simulink model "rigidBody2d"  (Simulink 7.5)
settings: Solver=ode45  StartTime=0.0  StopTime=40  RelTol=1e-3
undefined symbols (not defined in the file or in its folder): sigbuilder_block
settings Model: Creator=aaron  LastModifiedBy=aaron
settings DebuggingCC: SolverPrmCheckMsg=none

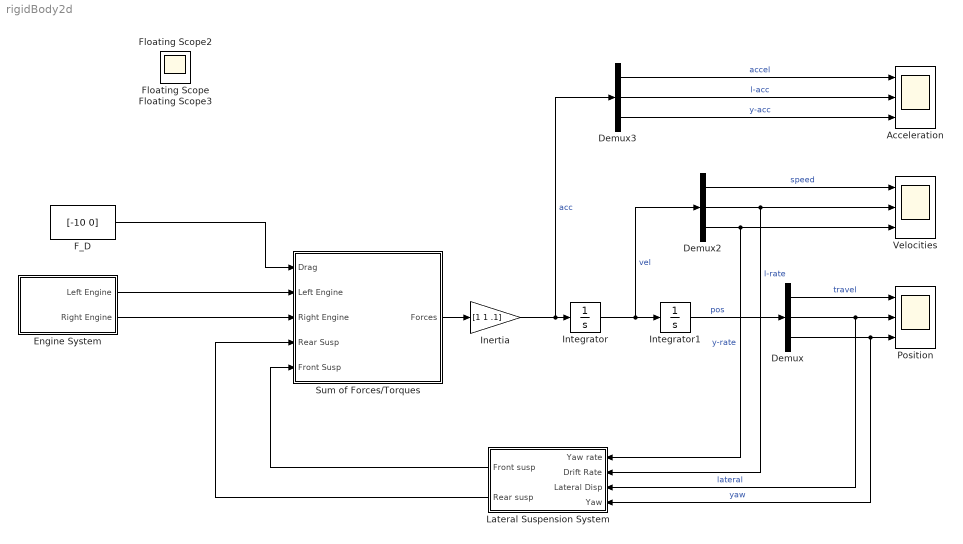
== system rigidBody2d ==
  Acceleration : Scope  NumInputPorts=3
      settings: YMin=-5~-5~-5  YMax=5~5~5  SaveName=position3
  Demux : Demux  Outputs=3
  Demux2 : Demux  Outputs=3
  Demux3 : Demux  Outputs=3
  Engine System : Subsystem
  F_D : Constant  Value=[-10 0]  OutDataType=fixdt(1, 16)  OutScaling=2^0
  Inertia : Gain  Gain=[1 1 .1]  ParameterDataType=fixdt(1, 16)  ParameterScaling=2^0  OutDataType=fixdt(1, 16)  OutScaling=2^0
  Integrator : Integrator  InitialCondition=[100 0 0]
  Integrator1 : Integrator  InitialCondition=[0 0 0]
  Lateral Suspension System : Subsystem
  Position : Scope  NumInputPorts=3
      settings: YMin=-5~-5~-5  YMax=5~5~5  SaveName=position
  Sum of Forces/Torques : Subsystem
  Velocities : Scope  NumInputPorts=3
      settings: YMin=-5~-5~-5  YMax=5~5~5  SaveName=position2
  Floating Scope : Scope
      settings: Floating=on
  Floating Scope2 : Scope
      settings: Floating=on  SaveName=ScopeData2
  Floating Scope3 : Scope
      settings: Floating=on  SaveName=ScopeData3
  wires:
  Integrator/1 -> Integrator1/1, Demux2/1  "vel"
  Inertia/1 -> Demux3/1, Integrator/1  "acc"
  Sum of Forces/Torques/1(Forces) -> Inertia/1
  Integrator1/1 -> Demux/1  "pos"
  Demux/1 -> Position/1  "travel"
  Demux/2 -> Position/2, Lateral Suspension System/3(Lateral Disp)  "lateral"
  Demux/3 -> Position/3, Lateral Suspension System/4(Yaw)  "yaw"
  Demux2/1 -> Velocities/1  "speed"
  Demux2/2 -> Velocities/2, Lateral Suspension System/2(Drift Rate)  "l-rate"
  Demux2/3 -> Velocities/3, Lateral Suspension System/1(Yaw rate)  "y-rate"
  Demux3/1 -> Acceleration/1  "accel"
  Demux3/2 -> Acceleration/2  "l-acc"
  Demux3/3 -> Acceleration/3  "y-acc"
  Engine System/1(Left Engine) -> Sum of Forces/Torques/2(Left Engine)
  Lateral Suspension System/1(Front susp) -> Sum of Forces/Torques/5(Front Susp)
  Lateral Suspension System/2(Rear susp) -> Sum of Forces/Torques/4(Rear Susp)
  F_D/1 -> Sum of Forces/Torques/1(Drag)
  Engine System/2(Right Engine) -> Sum of Forces/Torques/3(Right Engine)

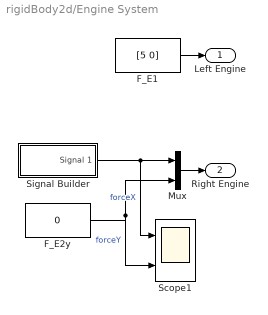
== system rigidBody2d/Engine System ==
  F_E1 : Constant  Value=[5 0]  OutDataType=fixdt(1, 16)  OutScaling=2^0
  F_E2y : Constant  Value=0  OutDataType=fixdt(1, 16)  OutScaling=2^0
  Mux : Mux  Inputs=2
  Scope1 : Scope  NumInputPorts=2
      settings: YMin=-5~-5  YMax=5~5  SaveName=engineErr
  Signal Builder : Subsystem  Tag=STV Subsys  LoadFcn=sigbuilder_block('load');  StartFcn=sigbuilder_block('start');  StopFcn=sigbuilder_block('stop');  ClipboardFcn=sigbuilder_block('clipboard');  mask(Sigbuilder block){}
      mask help: Create and generate interchangeable groups of signals whose waveforms are piecewise linear.
      mask init:
      | if ~strcmp(get_param(bdroot(gcbh),'SimulationStatus'),'stopped') tuvar = sigbuilder_block('maskInit'); end
      settings: CopyFcn=sigbuilder_block('copy');  DeleteFcn=sigbuilder_block('delete');  ModelCloseFcn=sigbuilder_block('modelClose');  PreSaveFcn=sigbuilder_block('preSave');  NameChangeFcn=sigbuilder_block('namechange');  OpenFcn=sigbuilder_block('open',[6 28.5 1428 717.75 ]);  CloseFcn=sigbuilder_block('close');
      mask Display: plot(0,0,100,100,[10,10,40,40,10],[80,20,20,80,80],[40,10],[50,50], [40,27,10],[65,72,56],[40,25,25,10],[28,28,43,43]);
  Left Engine : Outport
  Right Engine : Outport  Port=2
  wires:
  Signal Builder/1(Signal 1) -> Mux/1, Scope1/1  "forceX"
  F_E2y/1 -> Mux/2, Scope1/2  "forceY"
  F_E1/1 -> Left Engine/1
  Mux/1 -> Right Engine/1

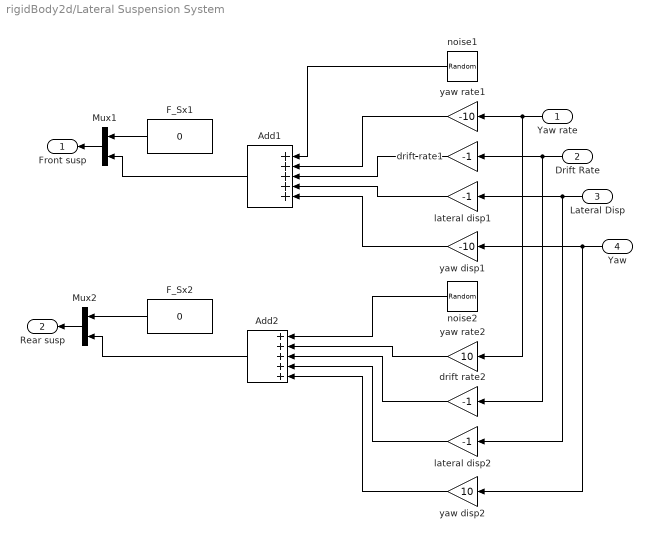
== system rigidBody2d/Lateral Suspension System ==
  Yaw rate : Inport
  Drift Rate : Inport  Port=2
  Lateral Disp : Inport  Port=3
  Yaw : Inport  Port=4
  Add1 : Sum  Inputs=+++++  OutDataType=fixdt(1, 16)  OutScaling=2^-10
  Add2 : Sum  Inputs=+++++  OutDataType=fixdt(1, 16)  OutScaling=2^-10
  F_Sx1 : Constant  Value=0  OutDataType=fixdt(1, 16)  OutScaling=2^0
  F_Sx2 : Constant  Value=0  OutDataType=fixdt(1, 16)  OutScaling=2^0
  Mux1 : Mux  Inputs=2
  Mux2 : Mux  Inputs=2
  drift rate1 : Gain  Gain=-1  ParameterDataType=fixdt(1, 16)  ParameterScaling=2^0  OutDataType=fixdt(1, 16)  OutScaling=2^0
  drift rate2 : Gain  Gain=-1  ParameterDataType=fixdt(1, 16)  ParameterScaling=2^0  OutDataType=fixdt(1, 16)  OutScaling=2^0
  lateral disp1 : Gain  Gain=-1  ParameterDataType=fixdt(1, 16)  ParameterScaling=2^0  OutDataType=fixdt(1, 16)  OutScaling=2^0
  lateral disp2 : Gain  Gain=-1  ParameterDataType=fixdt(1, 16)  ParameterScaling=2^0  OutDataType=fixdt(1, 16)  OutScaling=2^0
  noise1 : RandomNumber  Variance=.5  SampleTime=0.1
  noise2 : RandomNumber  Variance=.5  Seed=1  SampleTime=0.1
  yaw disp1 : Gain  Gain=-10  ParameterDataType=fixdt(1, 16)  ParameterScaling=2^0  OutDataType=fixdt(1, 16)  OutScaling=2^0
  yaw disp2 : Gain  Gain=10  ParameterDataType=fixdt(1, 16)  ParameterScaling=2^0  OutDataType=fixdt(1, 16)  OutScaling=2^0
  yaw rate1 : Gain  Gain=-10  ParameterDataType=fixdt(1, 16)  ParameterScaling=2^0  OutDataType=fixdt(1, 16)  OutScaling=2^0
  yaw rate2 : Gain  Gain=10  ParameterDataType=fixdt(1, 16)  ParameterScaling=2^0  OutDataType=fixdt(1, 16)  OutScaling=2^0
  Front susp : Outport
  Rear susp : Outport  Port=2
  wires:
  F_Sx1/1 -> Mux1/1
  Add1/1 -> Mux1/2
  F_Sx2/1 -> Mux2/1
  Add2/1 -> Mux2/2
  lateral disp1/1 -> Add1/4
  lateral disp2/1 -> Add2/4
  drift rate2/1 -> Add2/3
  drift rate1/1 -> Add1/3
  yaw disp2/1 -> Add2/5
  yaw disp1/1 -> Add1/5
  yaw rate2/1 -> Add2/2
  yaw rate1/1 -> Add1/2
  Yaw rate/1 -> yaw rate1/1, yaw rate2/1
  Drift Rate/1 -> drift rate1/1, drift rate2/1
  Lateral Disp/1 -> lateral disp1/1, lateral disp2/1
  Yaw/1 -> yaw disp1/1, yaw disp2/1
  Mux1/1 -> Front susp/1
  Mux2/1 -> Rear susp/1
  noise1/1 -> Add1/1
  noise2/1 -> Add2/1

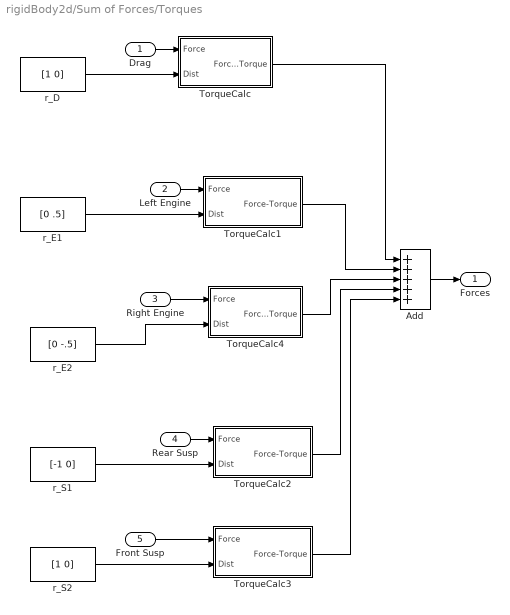
== system rigidBody2d/Sum of Forces/Torques ==
  Drag : Inport
  Left Engine : Inport  Port=2
  Right Engine : Inport  Port=3
  Rear Susp : Inport  Port=4
  Front Susp : Inport  Port=5
  Add : Sum  Inputs=+++++  OutDataType=fixdt(1, 16)  OutScaling=2^-10
  TorqueCalc : Subsystem
  TorqueCalc1 : Subsystem
  TorqueCalc2 : Subsystem
  TorqueCalc3 : Subsystem
  TorqueCalc4 : Subsystem
  r_D : Constant  Value=[1 0]  OutDataType=fixdt(1, 16)  OutScaling=2^0
  r_E1 : Constant  Value=[0 .5]  OutDataType=fixdt(1, 16)  OutScaling=2^0
  r_E2 : Constant  Value=[0 -.5]  OutDataType=fixdt(1, 16)  OutScaling=2^0
  r_S1 : Constant  Value=[-1 0]  OutDataType=fixdt(1, 16)  OutScaling=2^0
  r_S2 : Constant  Value=[1 0]  OutDataType=fixdt(1, 16)  OutScaling=2^0
  Forces : Outport
  wires:
  r_D/1 -> TorqueCalc/2(Dist)
  r_E1/1 -> TorqueCalc1/2(Dist)
  Drag/1 -> TorqueCalc/1(Force)
  Left Engine/1 -> TorqueCalc1/1(Force)
  r_S1/1 -> TorqueCalc2/2(Dist)
  Rear Susp/1 -> TorqueCalc2/1(Force)
  r_S2/1 -> TorqueCalc3/2(Dist)
  Add/1 -> Forces/1
  TorqueCalc3/1(Force-Torque) -> Add/5
  TorqueCalc2/1(Force-Torque) -> Add/4
  TorqueCalc1/1(Force-Torque) -> Add/2
  TorqueCalc/1(Force-Torque) -> Add/1
  Front Susp/1 -> TorqueCalc3/1(Force)
  Right Engine/1 -> TorqueCalc4/1(Force)
  r_E2/1 -> TorqueCalc4/2(Dist)
  TorqueCalc4/1(Force-Torque) -> Add/3

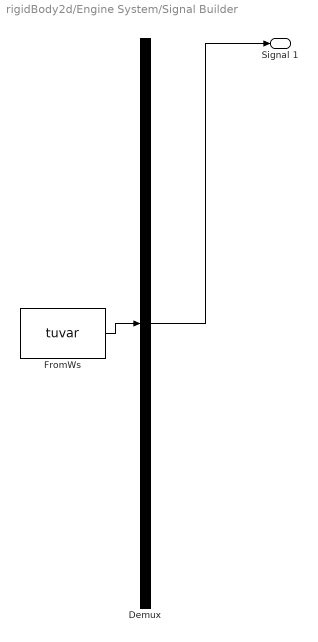
== system rigidBody2d/Engine System/Signal Builder ==
  Demux : Demux  Tag=STV Demux  Outputs=1
  FromWs : FromWorkspace  Tag=STV FromWs  VariableName=tuvar  SampleTime=0  SigBuilderData=DataTag0  VnvData=DataTag1
      SigBuilderData=|
      | common.afterFinalStr = 'Extrapolate'
      | common.sampleTime = 0
      | dataSet.timeRange = [0 40]
      | dataSet.name = 'Group 1'
      | sbobj.Groups.Name = 'Group 1'
      | sbobj.Groups.Signals.Name = 'Signal 1'
      | sbobj.Groups.Signals.XData = [0 1.24 1.24 4.1 4.1 12.88 12.88 15.14 15.14 18 40]
      | sbobj.Groups.Signals.YData = [5 5 6 6 5 5 1 1 5 5 2.5]
  Signal 1 : Outport  Tag=STV Outport  OutDataType=fixdt(1, 16)  OutScaling=2^0
  wires:
  Demux/1 -> Signal 1/1
  FromWs/1 -> Demux/1

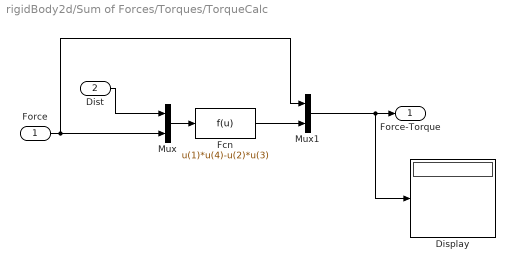
== system rigidBody2d/Sum of Forces/Torques/TorqueCalc ==
  Force : Inport
  Dist : Inport  Port=2
  Display : Display
  Fcn : Fcn  Expr=u(1)*u(4)-u(2)*u(3)
  Mux : Mux  Inputs=2
  Mux1 : Mux  Inputs=2
  Force-Torque : Outport
  wires:
  Force/1 -> Mux1/1, Mux/2
  Mux/1 -> Fcn/1
  Fcn/1 -> Mux1/2
  Mux1/1 -> Display/1, Force-Torque/1
  Dist/1 -> Mux/1

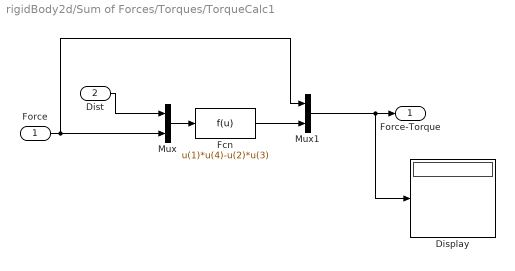
== system rigidBody2d/Sum of Forces/Torques/TorqueCalc1 ==
  Force : Inport
  Dist : Inport  Port=2
  Display : Display
  Fcn : Fcn  Expr=u(1)*u(4)-u(2)*u(3)
  Mux : Mux  Inputs=2
  Mux1 : Mux  Inputs=2
  Force-Torque : Outport
  wires:
  Force/1 -> Mux1/1, Mux/2
  Mux/1 -> Fcn/1
  Fcn/1 -> Mux1/2
  Mux1/1 -> Display/1, Force-Torque/1
  Dist/1 -> Mux/1

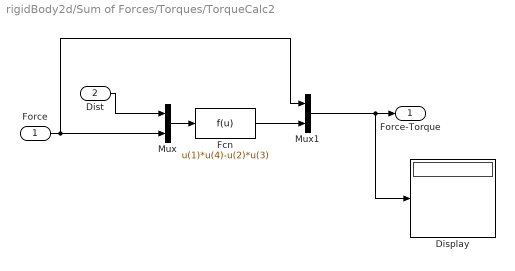
== system rigidBody2d/Sum of Forces/Torques/TorqueCalc2 ==
  Force : Inport
  Dist : Inport  Port=2
  Display : Display
  Fcn : Fcn  Expr=u(1)*u(4)-u(2)*u(3)
  Mux : Mux  Inputs=2
  Mux1 : Mux  Inputs=2
  Force-Torque : Outport
  wires:
  Force/1 -> Mux1/1, Mux/2
  Mux/1 -> Fcn/1
  Fcn/1 -> Mux1/2
  Mux1/1 -> Display/1, Force-Torque/1
  Dist/1 -> Mux/1

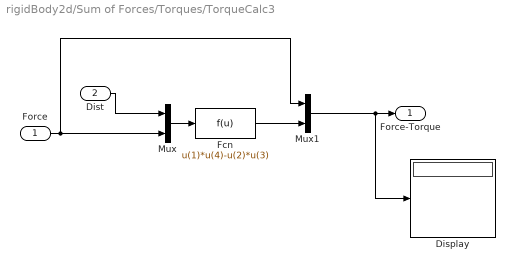
== system rigidBody2d/Sum of Forces/Torques/TorqueCalc3 ==
  Force : Inport
  Dist : Inport  Port=2
  Display : Display
  Fcn : Fcn  Expr=u(1)*u(4)-u(2)*u(3)
  Mux : Mux  Inputs=2
  Mux1 : Mux  Inputs=2
  Force-Torque : Outport
  wires:
  Force/1 -> Mux1/1, Mux/2
  Mux/1 -> Fcn/1
  Fcn/1 -> Mux1/2
  Mux1/1 -> Display/1, Force-Torque/1
  Dist/1 -> Mux/1

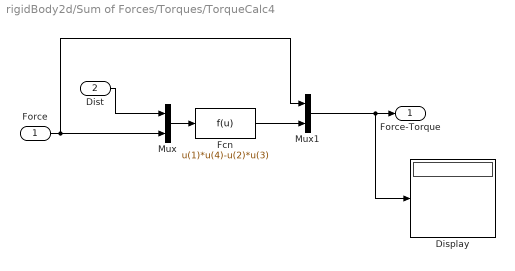
== system rigidBody2d/Sum of Forces/Torques/TorqueCalc4 ==
  Force : Inport
  Dist : Inport  Port=2
  Display : Display
  Fcn : Fcn  Expr=u(1)*u(4)-u(2)*u(3)
  Mux : Mux  Inputs=2
  Mux1 : Mux  Inputs=2
  Force-Torque : Outport
  wires:
  Force/1 -> Mux1/1, Mux/2
  Mux/1 -> Fcn/1
  Fcn/1 -> Mux1/2
  Mux1/1 -> Display/1, Force-Torque/1
  Dist/1 -> Mux/1
